simulink model "inversegeo"  (R2018a)
settings: Solver=VariableStepAuto  StartTime=0.0  StopTime=8  RelTol=1e-3
settings Model: Creator=ilyas  LastModifiedBy=ilyas

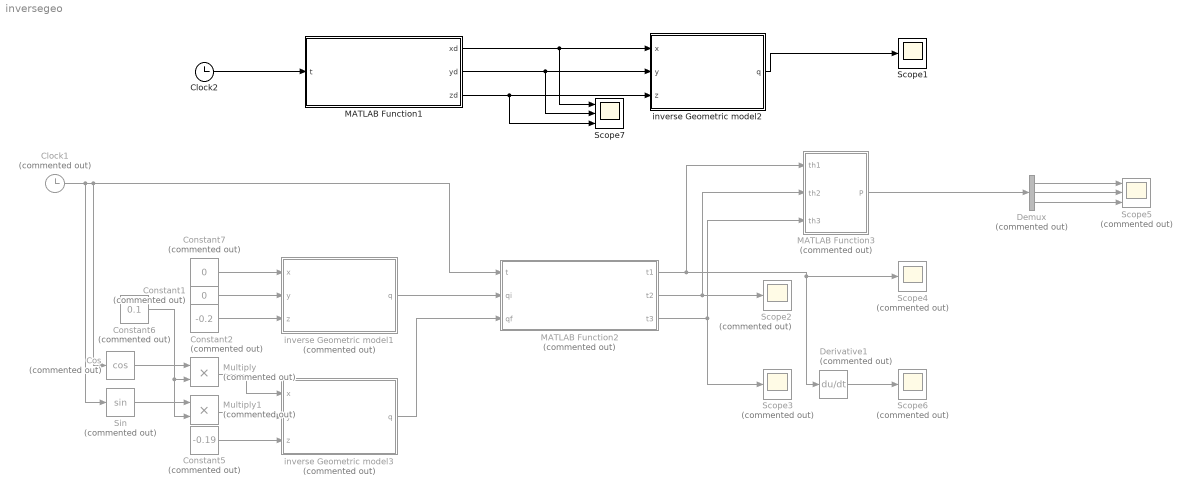
== system inversegeo ==
  Clock1 : Clock  Commented=on
  Clock2 : Clock
  Constant1 : Constant  Commented=on  Value=0
  Constant2 : Constant  Commented=on  Value=-0.2
  Constant5 : Constant  Commented=on  Value=-0.19
  Constant6 : Constant  Commented=on  Value=0.1
  Constant7 : Constant  Commented=on  Value=0
  Cos : Trigonometry  Commented=on  Operator=cos
  Demux : Demux  Commented=on  Outputs=3
  Derivative1 : Derivative  Commented=on
  MATLAB Function1 : MATLAB Function  TreatAsAtomicUnit=on
  MATLAB Function2 : MATLAB Function  Commented=on  TreatAsAtomicUnit=on
  MATLAB Function3 : MATLAB Function  Commented=on  TreatAsAtomicUnit=on
  Multiply : Product  Commented=on
  Multiply1 : Product  Commented=on
  Scope1 : Scope
  Scope{2..4,6} (4 alike) : Scope  Commented=on
  Scope5 : Scope  Commented=on  NumInputPorts=3
  Scope7 : Scope  NumInputPorts=3
  Sin : Trigonometry  Commented=on
  inverse Geometric model1 : MATLAB Function  Commented=on  TreatAsAtomicUnit=on
  inverse Geometric model2 : MATLAB Function  TreatAsAtomicUnit=on
  inverse Geometric model3 : MATLAB Function  Commented=on  TreatAsAtomicUnit=on
  wires:
  MATLAB Function1/2(yd) -> Scope7/2, inverse Geometric model2/2(y)
  MATLAB Function1/1(xd) -> Scope7/1, inverse Geometric model2/1(x)
  MATLAB Function2/1(t1) -> MATLAB Function3/1(th1), Derivative1/1, Scope4/1
  Derivative1/1 -> Scope6/1
  inverse Geometric model2/1(q) -> Scope1/1
  inverse Geometric model1/1(q) -> MATLAB Function2/2(qi)
  inverse Geometric model3/1(q) -> MATLAB Function2/3(qf)
  Multiply/1 -> inverse Geometric model3/1(x)
  Multiply1/1 -> inverse Geometric model3/2(y)
  Constant5/1 -> inverse Geometric model3/3(z)
  Constant2/1 -> inverse Geometric model1/3(z)
  Constant1/1 -> inverse Geometric model1/2(y)
  MATLAB Function2/2(t2) -> MATLAB Function3/2(th2), Scope2/1
  MATLAB Function2/3(t3) -> MATLAB Function3/3(th3), Scope3/1
  MATLAB Function3/1(P) -> Demux/1
  Demux/1 -> Scope5/1
  Demux/2 -> Scope5/2
  Demux/3 -> Scope5/3
  Clock1/1 -> MATLAB Function2/1(t), Cos/1, Sin/1
  Cos/1 -> Multiply/1
  Constant6/1 -> Multiply1/2, Multiply/2
  Constant7/1 -> inverse Geometric model1/1(x)
  Sin/1 -> Multiply1/1
  Clock2/1 -> MATLAB Function1/1(t)
  MATLAB Function1/3(zd) -> Scope7/3, inverse Geometric model2/3(z)

== matlab function inversegeo/inverse Geometric model2 ==
  data: x input; y input; z input; q output
function q  = inv_kin(x,y,z)
    
    sb= 0.415;%base equilateral triangle side
    sp= 0.086;%platform equilateral triangle side
    L=0.150;%upper legs length
    l = 0.3;
    wb=sb*sqrt(3)/6; 
    wp=sp*sqrt(3)/6; 
    up=sp*sqrt(3)/3; 
    
a   = wb - up;
b   = sp/2 - sqrt(3)/2*wb;
c   = wp - wb/2;
H   =[0;0;0];
G   = [0;0;0];
F   = [0;0;0];
t   = [0;0;0];
t1  = [0;0;0];
q   = [0;0;0];
q1  = [0;0;0];
dq  =  diff(q);
dq1 = diff(q1);
H(1) = 2*L*(y+a);
H(2) = -L*(sqrt(3)*(x+b) + y + c);
H(3) = L*(sqrt(3)*(x-b)-y-c);

G(1)= x^2 + y^2 + z^2 + a^2 + L^2 + 2*y*a -l^2;
G(2)= x^2 + y^2 + z^2 + b^2 + c^2 + L^2 + 2*(x*b+y*c) - l^2;
G(3)= x^2 + y^2 + z^2 + b^2 + c^2 + L^2 + 2*(-x*b+y*c) - l^2;

F(1)= 2*z*L;
F(2)= 2*z*L;
F(3)= 2*z*L;

for i = 1:3
    t(i) = (-F(i) + sqrt(H(i)^2 + F(i)^2 - G(i)^2))/(G(i)-H(i));
    q(i) = 2*atan(t(i));
    if q(i)<= 0 
        q(i) = 2*pi + q(i); 
        
    end

end

== matlab function inversegeo/inverse Geometric model1 ==
  data: x input; y input; z input; q output
function q  = inv_kin(x,y,z)
    
    sb= 0.415;%base equilateral triangle side
    sp= 0.086;%platform equilateral triangle side
    L=0.150;%upper legs length
    l = 0.2;
    wb=sb*sqrt(3)/6; 
    wp=sp*sqrt(3)/6; 
    up=sp*sqrt(3)/3; 
    
a   = wb - up;
b   = sp/2 - sqrt(3)/2*wb;
c   = wp - wb/2;
H   =[0;0;0];
G   = [0;0;0];
F   = [0;0;0];
t   = [0;0;0];
t1  = [0;0;0];
q   = [0;0;0];
q1  = [0;0;0];
dq  =  diff(q);
dq1 = diff(q1);
H(1) = 2*L*(y+a);
H(2) = -L*(sqrt(3)*(x+b) + y + c);
H(3) = L*(sqrt(3)*(x-b)-y-c);

G(1)= x^2 + y^2 + z^2 + a^2 + L^2 + 2*y*a -l^2;
G(2)= x^2 + y^2 + z^2 + b^2 + c^2 + L^2 + 2*(x*b+y*c) - l^2;
G(3)= x^2 + y^2 + z^2 + b^2 + c^2 + L^2 + 2*(-x*b+y*c) - l^2;

F(1)= 2*z*L;
F(2)= 2*z*L;
F(3)= 2*z*L;

for i = 1:3
    t(i) = (-F(i) + sqrt(H(i)^2 + F(i)^2 - G(i)^2))/(G(i)-H(i));
    q(i) = 2*atan(t(i));
    if q(i)<= 0 
        q(i) = 2*pi + q(i); 
        
    end

end

== matlab function inversegeo/MATLAB Function2 ==
  data: t input; t1 output; t2 output; t3 output; qi input; qf input
function [t1,t2,t3] = trj(t,qi,qf)
dqi = 0;
dqf = 0;
ti = 0;
tf = 0.1;
if t<tf
    t1=aubic(qi(1),qf(1),dqi,dqf,ti,tf,t);
    t2=aubic(qi(2),qf(2),dqi,dqf,ti,tf,t);
    t3=aubic(qi(3),qf(3),dqi,dqf,ti,tf,t);
else
    t1 = qf(1);
    t2 = qf(2);
    t3 = qf(3);
end
end

== matlab function inversegeo/inverse Geometric model3 ==
  data: x input; y input; z input; q output
function q  = inv_kin(x,y,z)
    
    sb= 0.415;%base equilateral triangle side
    sp= 0.086;%platform equilateral triangle side
    L=0.150;%upper legs length
    l = 0.2;
    wb=sb*sqrt(3)/6; 
    wp=sp*sqrt(3)/6; 
    up=sp*sqrt(3)/3; 
    
a   = wb - up;
b   = sp/2 - sqrt(3)/2*wb;
c   = wp - wb/2;
H   =[0;0;0];
G   = [0;0;0];
F   = [0;0;0];
t   = [0;0;0];
t1  = [0;0;0];
q   = [0;0;0];
q1  = [0;0;0];
dq  =  diff(q);
dq1 = diff(q1);
H(1) = 2*L*(y+a);
H(2) = -L*(sqrt(3)*(x+b) + y + c);
H(3) = L*(sqrt(3)*(x-b)-y-c);

G(1)= x^2 + y^2 + z^2 + a^2 + L^2 + 2*y*a -l^2;
G(2)= x^2 + y^2 + z^2 + b^2 + c^2 + L^2 + 2*(x*b+y*c) - l^2;
G(3)= x^2 + y^2 + z^2 + b^2 + c^2 + L^2 + 2*(-x*b+y*c) - l^2;

F(1)= 2*z*L;
F(2)= 2*z*L;
F(3)= 2*z*L;

for i = 1:3
    t(i) = (-F(i) + sqrt(H(i)^2 + F(i)^2 - G(i)^2))/(G(i)-H(i));
    q(i) = 2*atan(t(i));
    if q(i)<= 0 
        q(i) = 2*pi + q(i); 
        
    end

end

== matlab function inversegeo/MATLAB Function1 ==
  data: t input; xd output; yd output; zd output
function [xd,yd,zd] = trj(t)
zd = -0.2;
xd = 0;
yd = 0;
if t<2 
    yd = 0.15/2*t;
    xd = 0.15/2*t-0.15;
end
if t<4 && t>=2
    yd = -0.15/2*(t-2)+0.15;
    xd = 0.15/2*(t-2);
end
if t<6 && t>=4
    yd =  -0.15/2*(t-4);
    xd = -0.15/2*(t-4)+0.15;
end
if t<8 && t>=6
    yd = 0.15/2*(t-6)-0.15;
    xd = -0.15/2*(t-6);
end
end

== matlab function inversegeo/MATLAB Function3 ==
  data: th1 input; P output; th2 input; th3 input
function P  = fpk( th1,th2,th3 )
sb= 0.415;%base equilateral triangle side
    sp= 0.086;%platform equilateral triangle side
    L=0.150;%upper legs length
    l = 0.200;
    wb=sb*sqrt(3)/6; 
    wp=sp*sqrt(3)/6; 
    up=sp*sqrt(3)/3; 

    %Representation of E1, E2, E3 in the fixed base frame
    e1=[(wb-up)+L*cos(th1) 0 -L*sin(th1)];
    e2=[(wb-up)+L*cos(th2) 0 -L*sin(th2)];
    e3=[(wb-up)+L*cos(th3) 0 -L*sin(th3)];
    E1=rot_0Z(0)*e1';
    E2=rot_0Z(2*pi/3)*e2'; 
    E3=rot_0Z(4*pi/3)*e3';
    %calculation of cartisien position using steps of sec(2.4)
    M=[E1';E2';E3'];
    M1=-M;
    N=zeros(2,3);
    V=zeros(2);
    for i=1:2
        for j=1:3
            N(i,j)=2*(M1(1,j)-M1(i+1,j));
        end
        V(i)=((M1(i+1,1)^2+M1(i+1,2)^2+M1(i+1,3)^2)-...
            (M1(1,1)^2+M1(1,2)^2+M1(1,3)^2));
    end
    
    D=N(1,1)*N(2,2)-N(2,1)*N(1,2);
    f1=(N(2,2)*V(1)-N(1,2)*V(2))/D;
    f2=(N(1,1)*V(2)-N(2,1)*V(1))/D;
    f3=(N(1,2)*N(2,3)-N(1,3)*N(2,2))/D;%fx
    f4=(N(2,1)*N(1,3)-N(1,1)*N(2,3))/D;%fy
    E=(f3^2 + f4^2 + 1);
    F=(2*M1(3,3) + 2*f3*(f1 + M1(3,1)) + 2*f4*(f2 + M1(3,2)));
    G=(f1 + M1(3,1))^2 + (f2 + M1(3,2))^2 + M1(3,3)^2-l^2;
    d = F^2-4*E*G;
    if d < 0
        z = nan;
        x = nan;
        y = nan;
        S = -1;
    else
        z=(-F-sqrt(d))/(2*E);
        x=f1+f3*z;
        y=f2+f4*z;
        if (z == 0)&&(x==0)&&(y==0)
            S = -1;
        else 
            S=0;
        end
    end
    P=[x;y;z];
    P=rot_0Z(-pi/2)*P;
   
end
